simulink model "SimulinkLR2"  (R2016a)
settings: Solver=VariableStepAuto  StartTime=0.0  StopTime=10E-2  RelTol=1e-3
values from neighbouring files (symbols this model uses):
  A = 0.5E-3    (= 0.0005)    [LR2.m]
  N = 1000    [LR2.m]
  T = 10E-3    (= 0.01)    [LR2.m]
undefined symbols (not defined in the file or in its folder): DiscIntNeverNeededParam
libraries: dspsrcs4 x1
settings Model: Creator=Энверыч  LastModifiedBy=Энверыч

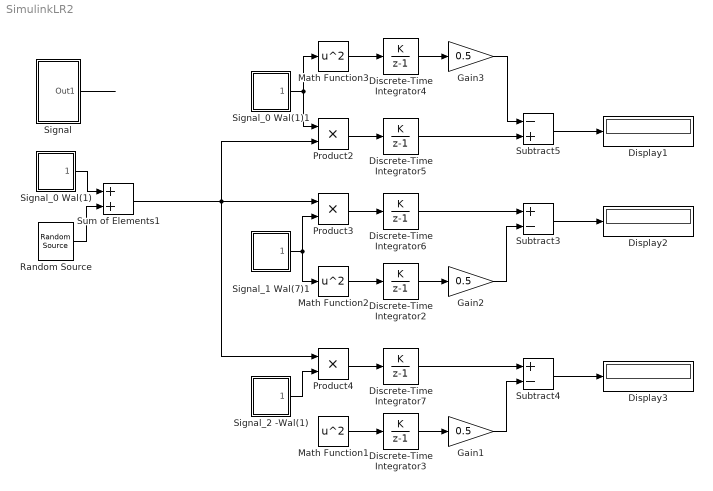
== system SimulinkLR2 ==
  Discrete-Time Integrator{2..7} (6 alike) : DiscreteIntegrator  IntegratorMethod=Accumulation: Forward Euler  InitialConditionSetting=State (most efficient)  SampleTime=T/N  ICPrevOutput=DiscIntNeverNeededParam  ICPrevScaledInput=DiscIntNeverNeededParam
  Display1 : Display
  Display2 : Display
  Display3 : Display
  Gain1 : Gain  Gain=0.5
  Gain2 : Gain  Gain=0.5
  Gain3 : Gain  Gain=0.5
  Math Function1 : Math  Operator=square  SaturateOnIntegerOverflow=on
  Math Function2 : Math  Operator=square  SaturateOnIntegerOverflow=on
  Math Function3 : Math  Operator=square  SaturateOnIntegerOverflow=on
  Product2 : Product
  Product3 : Product
  Product4 : Product
  Random Source : dspsrcs4/Random Source  SrcType=Uniform  NormMethod=Ziggurat  CltLength=12  MinVal=0  MaxVal=1  MeanVal=0  VarVal=1  RepMode=Not repeatable  rawSeed=1  IsInherit=off  SampMode=Discrete  SampTime=1  SampFrame=1  DataType=Double  OutComplex=Real  OutputFrames=off
  "Signal " : Subsystem
  Signal_0 Wal(1) : Subsystem
  Signal_0 Wal(1)1 : Subsystem
  Signal_1 Wal(7)1 : Subsystem
  Signal_2 -Wal(1) : Subsystem
  Subtract3 : Sum  Inputs=+-
  Subtract4 : Sum  Inputs=+-
  Subtract5 : Sum  Inputs=-+
  Sum of Elements1 : Sum
  wires:
  Signal_0 Wal(1)/1(Out1) -> Sum of Elements1/1
  Random Source/1 -> Sum of Elements1/2
  "Signal "/1(Out1) -> ?
  Product2/1 -> Discrete-Time Integrator5/1
  Discrete-Time Integrator5/1 -> Subtract5/2
  Product3/1 -> Discrete-Time Integrator6/1
  Discrete-Time Integrator6/1 -> Subtract3/1
  Product4/1 -> Discrete-Time Integrator7/1
  Discrete-Time Integrator7/1 -> Subtract4/1
  Signal_0 Wal(1)1/1(Out1) -> Product2/1, Math Function3/1
  Sum of Elements1/1 -> Product4/1, Product3/1, Product2/2
  Signal_2 -Wal(1)/1(Out1) -> Product4/2
  Discrete-Time Integrator3/1 -> Gain1/1
  Math Function1/1 -> Discrete-Time Integrator3/1
  Signal_1 Wal(7)1/1(Out1) -> Product3/2, Math Function2/1
  Math Function3/1 -> Discrete-Time Integrator4/1
  Discrete-Time Integrator4/1 -> Gain3/1
  Math Function2/1 -> Discrete-Time Integrator2/1
  Discrete-Time Integrator2/1 -> Gain2/1
  Gain2/1 -> Subtract3/2
  Gain1/1 -> Subtract4/2
  Gain3/1 -> Subtract5/1
  Subtract5/1 -> Display1/1
  Subtract3/1 -> Display2/1
  Subtract4/1 -> Display3/1

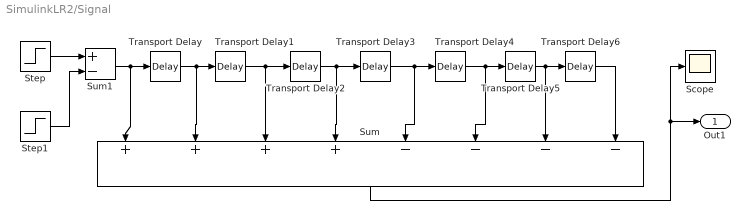
== system SimulinkLR2/Signal  ==
  Scope : Scope
  Step : Step  Time=0  After=A  SampleTime=0
  Step1 : Step  Time=T  After=A  SampleTime=0
  Sum : Sum  Inputs=++++----
  Sum1 : Sum  Inputs=+-
  Transport Delay{,1..6} (7 alike) : TransportDelay  DelayTime=T
  Out1 : Outport
  wires:
  Step1/1 -> Sum1/2
  Transport Delay5/1 -> Transport Delay6/1, Sum/7
  Transport Delay4/1 -> Sum/6, Transport Delay5/1
  Transport Delay/1 -> Sum/2, Transport Delay1/1
  Transport Delay2/1 -> Sum/4, Transport Delay3/1
  Transport Delay6/1 -> Sum/8
  Sum/1 -> Out1/1, Scope/1
  Step/1 -> Sum1/1
  Transport Delay3/1 -> Sum/5, Transport Delay4/1
  Transport Delay1/1 -> Sum/3, Transport Delay2/1
  Sum1/1 -> Transport Delay/1, Sum/1

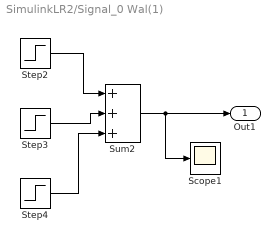
== system SimulinkLR2/Signal_0 Wal(1) ==
  Scope1 : Scope
  Step2 : Step  Time=0  After=A  SampleTime=0
  Step3 : Step  Time=4*T  After=-2*A  SampleTime=0
  Step4 : Step  Time=8*T  After=A  SampleTime=0
  Sum2 : Sum  Inputs=+++
  Out1 : Outport
  wires:
  Sum2/1 -> Out1/1, Scope1/1
  Step4/1 -> Sum2/3
  Step3/1 -> Sum2/2
  Step2/1 -> Sum2/1

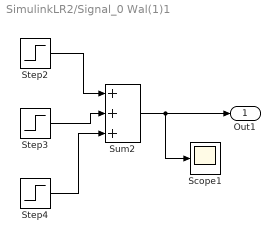
== system SimulinkLR2/Signal_0 Wal(1)1 ==
  Scope1 : Scope
  Step2 : Step  Time=0  After=A  SampleTime=0
  Step3 : Step  Time=4*T  After=-2*A  SampleTime=0
  Step4 : Step  Time=8*T  After=A  SampleTime=0
  Sum2 : Sum  Inputs=+++
  Out1 : Outport
  wires:
  Sum2/1 -> Out1/1, Scope1/1
  Step4/1 -> Sum2/3
  Step3/1 -> Sum2/2
  Step2/1 -> Sum2/1

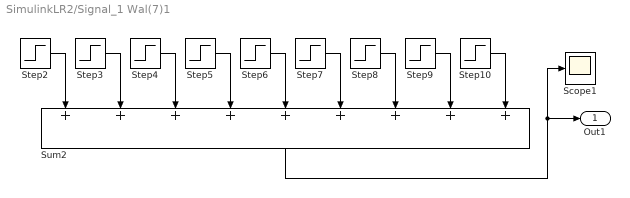
== system SimulinkLR2/Signal_1 Wal(7)1 ==
  Scope1 : Scope
  Step10 : Step  Time=8*T  After=A  SampleTime=0
  Step2 : Step  Time=0  After=A  SampleTime=0
  Step3 : Step  Time=T  After=-2*A  SampleTime=0
  Step4 : Step  Time=2*T  After=2*A  SampleTime=0
  Step5 : Step  Time=3*T  After=-2*A  SampleTime=0
  Step6 : Step  Time=4*T  After=2*A  SampleTime=0
  Step7 : Step  Time=5*T  After=-2*A  SampleTime=0
  Step8 : Step  Time=6*T  After=2*A  SampleTime=0
  Step9 : Step  Time=7*T  After=-2*A  SampleTime=0
  Sum2 : Sum  Inputs=+++++++++
  Out1 : Outport
  wires:
  Sum2/1 -> Out1/1, Scope1/1
  Step3/1 -> Sum2/2
  Step10/1 -> Sum2/9
  Step7/1 -> Sum2/6
  Step8/1 -> Sum2/7
  Step6/1 -> Sum2/5
  Step9/1 -> Sum2/8
  Step5/1 -> Sum2/4
  Step4/1 -> Sum2/3
  Step2/1 -> Sum2/1

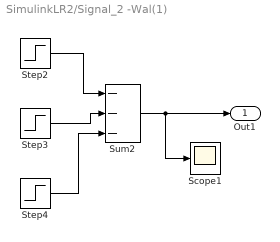
== system SimulinkLR2/Signal_2 -Wal(1) ==
  Scope1 : Scope
  Step2 : Step  Time=0  After=A  SampleTime=0
  Step3 : Step  Time=4*T  After=-2*A  SampleTime=0
  Step4 : Step  Time=8*T  After=A  SampleTime=0
  Sum2 : Sum  Inputs=---
  Out1 : Outport
  wires:
  Sum2/1 -> Out1/1, Scope1/1
  Step4/1 -> Sum2/3
  Step3/1 -> Sum2/2
  Step2/1 -> Sum2/1
